simulink model "part2_MAIN_2019_ayonnn"  (R2023b)
settings: Solver=FixedStepAuto  StartTime=0.0  StopTime=8000  FixedStep=0.1  RelTol=1e-3
values from neighbouring files (symbols this model uses):
  Af = diag(ti)    [init.m]    (also in init_old.m)
  Aw = [zeros(3) eye(3) ... (first row only)    [get_observer_parameters.m]
  B = [thr1 thr2_x thr2_y thr3 thr4_x thr4_y thr5_x thr5_y]    [B_redistributed.m]    (also in check_alg.m = [1 2 3 4 5 6 7 8; get_observer_parameters.m = [zeros(6,3);zeros(3,3);zeros(3,3);inv(M)])
  change_position_time = 1200    [init.m]    (also in init_old.m)
  Cw = [zeros(3) eye(3)]    [get_observer_parameters.m]
  D = Damping    [init.m]    (also in init_old.m)
  Damping = diag([2.6486e5, 8.8164e5, 3.3774e8])    [init.m]    (also in init_old.m)
  direction_limit = pi/36    (= 0.0872664625997)    [init.m]    (also in init_old.m)
  direction_time_constant = 100    [init.m]    (also in init_old.m)
  dt = 0.1    [get_observer_parameters.m]
  E = [Ew, zeros(6,3) ... (first row only)    [get_observer_parameters.m]
  Gamma = diag(omega_is)    [init.m]    (also in init_old.m)
  gust_limit = 40    [init.m]    (also in init_old.m)
  H = [Cw, eye(3), zeros(3,3) zeros(3,3)]    [get_observer_parameters.m]    (also in quadprog.m = 2*diag([w.' w.' q.' q.' w_alpha.' w_alpha.']); quadprog_basic.m = 2*diag([w.' w.' q.' q.']); quadprog_false.m = 2*diag([w.' w.' q.' q.' w_alpha.' w_alpha.']))
  height = 3    [init.m]    (also in init_old.m)
  inv_M = inv(M)    [get_observer_parameters.m]
  inv_Tb = inv(Tb)    [get_observer_parameters.m]
  kappa = 0.003    [init.m]    (also in init_old.m)
  kappa2 = 0.0026    [init.m]    (also in init_old.m)
  Kd = [1660451.40544401; 3920391.80535684; 1605063439.04156]    [init.m]    (also in init_old.m)
  Ki = [137.081306245593; 3163.274947400198; 335358.448218978]    [init.m]    (also in init_old.m)
  Kp = [75459.3345349083; 277551.73586971; 120744473.878042]    [init.m]    (also in init_old.m)
  L = 1800    [init.m]    (also in init_old.m)
  M = Mass    [init.m]    (also in init_old.m)
  mean_wind_direction = pi    (= 3.14159265359)    [init.m]    (also in init_old.m)
  observer_type = 1    [init.m]    (also in init_old.m = 0)
  Omega = diag([omega_n, omega_n, omega_n])    [get_observer_parameters.m]    (also in init.m = diag(2*omega_is.*zeta_is); init_old.m = diag(2*omega_is.*zeta_is))
  Q = diag([0.1,0.1,pi/180,1e6,1e6,1e9])*10e3    [get_observer_parameters.m]
  R = diag([1,0.1,0.1*pi/180])*10e-3    [get_observer_parameters.m]
  simulation = 2    [init.m]    (also in init_old.m = 1)
  slow_varying_limit = 1    [init.m]    (also in init_old.m)
  slow_varying_time_constant = 100    [init.m]    (also in init_old.m)
  TAU = dt*E    [get_observer_parameters.m]
  Tb = 0.1 * eye(3)    [get_observer_parameters.m]
  u10 = 12    [init.m]    (also in init_old.m)
  vessel =     [test.mat]
  wind = 1    [init.m]    (also in init_old.m)
undefined symbols (not defined in the file or in its folder): Hoerner, ModelParams, npf, Param, thrusters, WaveModel
libraries: simulink x10, slpidlib x6, dspsigops x6, marine_hydro x4, marine_gnc x2
(part 2 of 3)

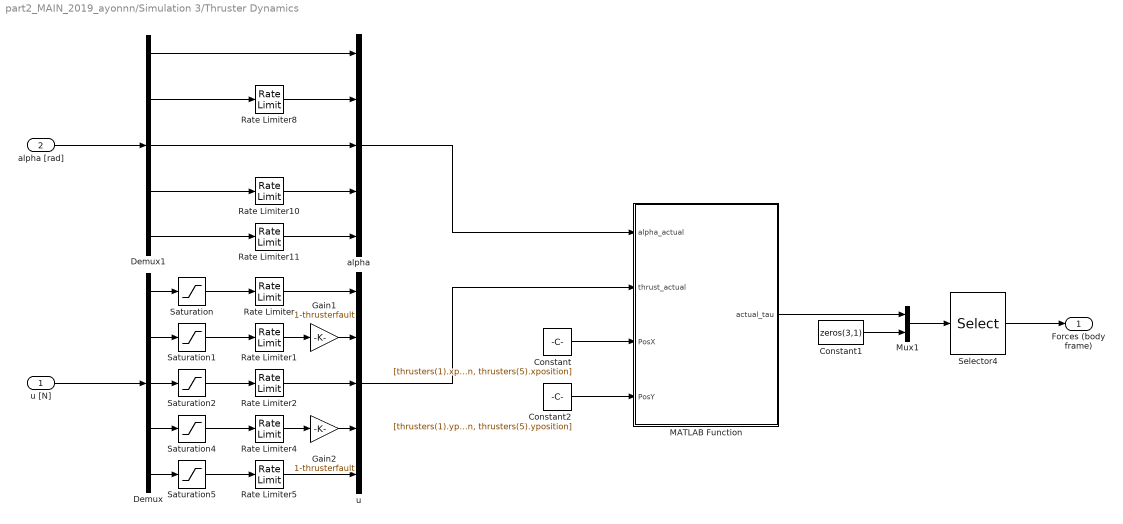
== system part2_MAIN_2019_ayonnn/Simulation 3/Thruster Dynamics ==
  u [N] : Inport
  alpha [rad] : Inport  Port=2
  Constant : Constant  Value=[thrusters(1).xposition, thrusters(2).xposition, thrusters(3).xposition, thrusters(4).xposition, thrusters(5).xposition]
  Constant1 : Constant  Value=zeros(3,1)
  Constant2 : Constant  Value=[thrusters(1).yposition, thrusters(2).yposition, thrusters(3).yposition, thrusters(4).yposition, thrusters(5).yposition]
  Demux : Demux  Outputs=5
  Demux1 : Demux  Outputs=5
  Gain1 : Gain  Gain=1-thrusterfault
  Gain2 : Gain  Gain=1-thrusterfault
  MATLAB Function : MATLAB Function  TreatAsAtomicUnit=on
  Mux1 : Mux  Inputs=2
  Rate Limiter : RateLimiter  RisingSlewLimit=thrusters(1).rate  FallingSlewLimit=-thrusters(1).rate  SampleTimeMode=inherited
  Rate Limiter1 : RateLimiter  RisingSlewLimit=thrusters(2).rate  FallingSlewLimit=-thrusters(2).rate  SampleTimeMode=inherited
  Rate Limiter10 : RateLimiter  RisingSlewLimit=thrusters(4).rotationspeed  FallingSlewLimit=-thrusters(4).rotationspeed  SampleTimeMode=inherited
  Rate Limiter11 : RateLimiter  RisingSlewLimit=thrusters(5).rotationspeed  FallingSlewLimit=-thrusters(5).rotationspeed  SampleTimeMode=inherited
  Rate Limiter2 : RateLimiter  RisingSlewLimit=thrusters(3).rate  FallingSlewLimit=-thrusters(3).rate  SampleTimeMode=inherited
  Rate Limiter4 : RateLimiter  RisingSlewLimit=thrusters(4).rate  FallingSlewLimit=-thrusters(4).rate  SampleTimeMode=inherited
  Rate Limiter5 : RateLimiter  RisingSlewLimit=thrusters(5).rate  FallingSlewLimit=-thrusters(5).rate  SampleTimeMode=inherited
  Rate Limiter8 : RateLimiter  RisingSlewLimit=thrusters(2).rotationspeed  FallingSlewLimit=-thrusters(2).rotationspeed  SampleTimeMode=inherited
  Saturation : Saturate  UpperLimit=thrusters(1).thrust  LowerLimit=-thrusters(1).thrust
  Saturation1 : Saturate  UpperLimit=thrusters(2).thrust  LowerLimit=-thrusters(2).thrust
  Saturation2 : Saturate  UpperLimit=thrusters(3).thrust  LowerLimit=-thrusters(3).thrust
  Saturation4 : Saturate  UpperLimit=thrusters(4).thrust  LowerLimit=-thrusters(4).thrust
  Saturation5 : Saturate  UpperLimit=thrusters(5).thrust  LowerLimit=-thrusters(5).thrust
  Selector4 : Selector  InputPortWidth=6  IndexOptions=Index vector (dialog)  Indices=[1 2 4 5 6 3]  OutputSizes=1
  alpha : Mux  Inputs=5
  u : Mux  Inputs=5
  "Forces (body frame) " : Outport  VectorParamsAs1DForOutWhenUnconnected=off
  wires:
  Rate Limiter2/1 -> u/3
  Saturation/1 -> Rate Limiter/1
  Mux1/1 -> Selector4/1
  Constant1/1 -> Mux1/2
  Saturation4/1 -> Rate Limiter4/1
  Demux/2 -> Saturation1/1
  Saturation1/1 -> Rate Limiter1/1
  Demux/1 -> Saturation/1
  Demux/3 -> Saturation2/1
  Saturation2/1 -> Rate Limiter2/1
  Selector4/1 -> "Forces (body frame) "/1
  Gain1/1 -> u/2
  Rate Limiter1/1 -> Gain1/1
  Rate Limiter/1 -> u/1
  Rate Limiter4/1 -> Gain2/1
  Saturation5/1 -> Rate Limiter5/1
  u [N]/1 -> Demux/1
  alpha [rad]/1 -> Demux1/1
  Constant/1 -> MATLAB Function/3(PosX)
  Constant2/1 -> MATLAB Function/4(PosY)
  u/1 -> MATLAB Function/2(thrust_actual)
  alpha/1 -> MATLAB Function/1(alpha_actual)
  MATLAB Function/1(actual_tau) -> Mux1/1
  Rate Limiter10/1 -> alpha/4
  Demux1/4 -> Rate Limiter10/1
  Demux1/5 -> Rate Limiter11/1
  Rate Limiter11/1 -> alpha/5
  Demux1/1 -> alpha/1
  Gain2/1 -> u/4
  Demux/4 -> Saturation4/1
  Demux/5 -> Saturation5/1
  Rate Limiter5/1 -> u/5
  Demux1/2 -> Rate Limiter8/1
  Rate Limiter8/1 -> alpha/2
  Demux1/3 -> alpha/3

== system part2_MAIN_2019_ayonnn/Simulation 3/Wave ==
  eta : Inport
  waves : Inport  Port=2
  Gain : Gain  Gain=waveforces
  Sum : Sum
  Wave loads (U=0) : marine_hydro/Hydro Library/Wave loads (U=0)  SystemSampleTime=-1  VariantActivationTime=update diagram  AllowFlexibleInterface=on  Latency=0  AutoFrameSizeCalculation=off
      settings: SourceProductName=MSS Hydro
  Wave : Outport  VectorParamsAs1DForOutWhenUnconnected=off
  wires:
  eta/1 -> Wave loads (U=0)/1
  waves/1 -> Wave loads (U=0)/2
  Sum/1 -> Gain/1
  Wave loads (U=0)/1 -> Sum/1
  Wave loads (U=0)/2 -> Sum/2
  Gain/1 -> Wave/1

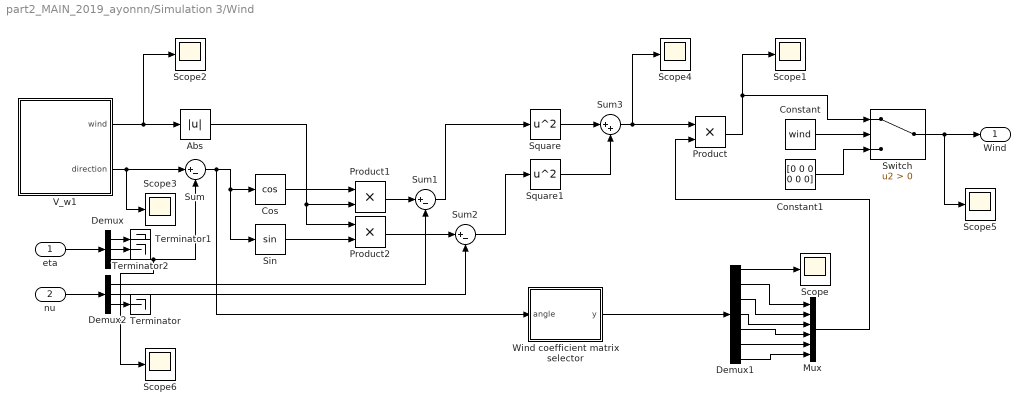
== system part2_MAIN_2019_ayonnn/Simulation 3/Wind ==
  eta : Inport
  nu : Inport  Port=2
  Abs : Abs  SaturateOnIntegerOverflow=off
  Constant : Constant  Value=wind
  Constant1 : Constant  Value=[0 0 0 0 0 0]
  Cos : Trigonometry  Operator=cos
  Demux : Demux  Outputs=3
  Demux1 : Demux  Outputs=7
  Demux2 : Demux  Outputs=3
  Mux : Mux  Inputs=6
  Product : Product
  Product1 : Product
  Product2 : Product
  Scope{,1..6} (7 alike) : Scope
  Sin : Trigonometry
  Square : Math  Operator=square  SignedPower=on
  Square1 : Math  Operator=square  SignedPower=on
  Sum : Sum  Inputs=|+-
  Sum1 : Sum  Inputs=|+-
  Sum2 : Sum  Inputs=|+-
  Sum3 : Sum  Inputs=|++
  Switch : Switch  Criteria=u2 > Threshold  SaturateOnIntegerOverflow=off  InputSameDT=off
  Terminator : Terminator
  Terminator1 : Terminator
  Terminator2 : Terminator
  V_w1 : Subsystem
  Wind coefficient matrix selector : MATLAB Function  TreatAsAtomicUnit=on
  Wind : Outport  VectorParamsAs1DForOutWhenUnconnected=off
  wires:
  V_w1/1(wind) -> Scope2/1, Abs/1
  Abs/1 -> Product2/1, Product1/2
  eta/1 -> Demux/1
  V_w1/2(direction) -> Scope3/1, Sum/1
  Demux/3 -> Scope6/1, Sum/2
  Wind coefficient matrix selector/1(y) -> Demux1/1
  Demux1/1 -> Scope/1
  Demux1/2 -> Mux/1
  Demux1/3 -> Mux/2
  Demux1/4 -> Mux/3
  Demux1/5 -> Mux/4
  Demux1/6 -> Mux/5
  Demux1/7 -> Mux/6
  Product/1 -> Switch/1, Scope1/1
  Mux/1 -> Product/2
  Sum/1 -> Wind coefficient matrix selector/1(angle), Sin/1, Cos/1
  nu/1 -> Demux2/1
  Sin/1 -> Product2/2
  Cos/1 -> Product1/1
  Product1/1 -> Sum1/1
  Product2/1 -> Sum2/1
  Demux2/1 -> Sum1/2
  Demux2/2 -> Sum2/2
  Sum1/1 -> Square/1
  Sum2/1 -> Square1/1
  Sum3/1 -> Scope4/1, Product/1
  Square/1 -> Sum3/1
  Square1/1 -> Sum3/2
  Demux2/3 -> Terminator/1
  Demux/1 -> Terminator1/1
  Demux/2 -> Terminator2/1
  Switch/1 -> Scope5/1, Wind/1
  Constant/1 -> Switch/2
  Constant1/1 -> Switch/3

== system part2_MAIN_2019_ayonnn/Original/Current (North - East)/Subsystem ==
  Mux1 : Mux  Inputs=3
  Scope : Scope
  Step1 : Step  Time=0  After=0  SampleTime=0
  Step2 : Step  Time=0  After=-0.2  SampleTime=0
  Step3 : Step  Time=0  After=0  SampleTime=0
  Out1 : Outport
  wires:
  Mux1/1 -> Scope/1, Out1/1
  Step1/1 -> Mux1/1
  Step2/1 -> Mux1/2
  Step3/1 -> Mux1/3

== system part2_MAIN_2019_ayonnn/Original/Current (North - East)/Subsystem1 ==
  Add : Sum  Inputs=+++
  Cos : Trigonometry  Operator=cos
  Gain : Gain  Gain=pi/180
  Matrix Multiply : Product
  Matrix Multiply1 : Product
  Mux : Mux  Inputs=3
  Ramp : simulink/Sources/Ramp  slope=0.45  start=2  InitialOutput=0
  Ramp1 : simulink/Sources/Ramp  slope=-0.45  start=202  InitialOutput=0
  Scope : Scope  NumInputPorts=3
  Sin : Trigonometry
  Step : Step  Time=2  After=0.5  SampleTime=0
  Step1 : Step  Time=2  Before=180  After=180  SampleTime=0
  Step2 : Step  Time=0  After=0  SampleTime=0
  Out1 : Outport
  wires:
  Step1/1 -> Add/1
  Ramp/1 -> Add/2
  Ramp1/1 -> Add/3
  Step/1 -> Matrix Multiply1/1, Matrix Multiply/1
  Sin/1 -> Matrix Multiply1/2, Scope/1
  Cos/1 -> Matrix Multiply/2, Scope/2
  Matrix Multiply/1 -> Mux/1
  Matrix Multiply1/1 -> Mux/2
  Step2/1 -> Mux/3
  Mux/1 -> Scope/3, Out1/1
  Add/1 -> Gain/1
  Gain/1 -> Sin/1, Cos/1

== system part2_MAIN_2019_ayonnn/Original/Current (North - East)/Subsystem2 ==
  Mux : Mux  Inputs=3
  Step : Step  Time=0  After=0  SampleTime=0
  Out1 : Outport
  wires:
  Mux/1 -> Out1/1
  Step/1 -> Mux/3, Mux/2, Mux/1

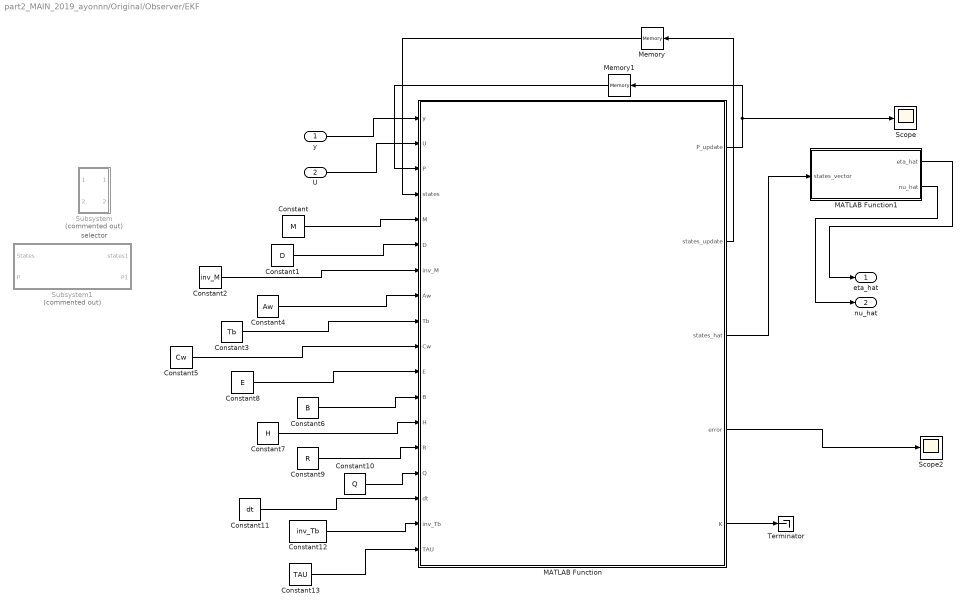
== system part2_MAIN_2019_ayonnn/Original/Observer/EKF ==
  note: selector
  y : Inport
  U : Inport  Port=2
  Constant : Constant  Value=M
  Constant1 : Constant  Value=D
  Constant10 : Constant  Value=Q
  Constant11 : Constant  Value=dt
  Constant12 : Constant  Value=inv_Tb
  Constant13 : Constant  Value=TAU
  Constant2 : Constant  Value=inv_M
  Constant3 : Constant  Value=Tb
  Constant4 : Constant  Value=Aw
  Constant5 : Constant  Value=Cw
  Constant6 : Constant  Value=B
  Constant7 : Constant  Value=H
  Constant8 : Constant  Value=E
  Constant9 : Constant  Value=R
  MATLAB Function : MATLAB Function  TreatAsAtomicUnit=on
  MATLAB Function1 : MATLAB Function  TreatAsAtomicUnit=on
  Memory : Memory  InitialCondition=zeros(15,1)
  Memory1 : Memory  InitialCondition=eye(15,15)
  Scope : Scope
  Scope2 : Scope
  Subsystem : Subsystem  Commented=on
  Subsystem1 : Subsystem  Commented=on
  Terminator : Terminator
  eta_hat : Outport
  nu_hat : Outport  Port=2
  wires:
  U/1 -> MATLAB Function/2(U)
  MATLAB Function1/1(eta_hat) -> eta_hat/1
  MATLAB Function/3(states_hat) -> MATLAB Function1/1(states_vector)
  MATLAB Function/4(error) -> Scope2/1
  y/1 -> MATLAB Function/1(y)
  MATLAB Function1/2(nu_hat) -> nu_hat/1
  MATLAB Function/2(states_update) -> Memory/1
  Constant/1 -> MATLAB Function/5(M)
  Constant1/1 -> MATLAB Function/6(D)
  Constant2/1 -> MATLAB Function/7(inv_M)
  Constant4/1 -> MATLAB Function/8(Aw)
  Constant3/1 -> MATLAB Function/9(Tb)
  Constant5/1 -> MATLAB Function/10(Cw)
  Constant8/1 -> MATLAB Function/11(E)
  Constant6/1 -> MATLAB Function/12(B)
  Constant7/1 -> MATLAB Function/13(H)
  Constant9/1 -> MATLAB Function/14(R)
  Constant10/1 -> MATLAB Function/15(Q)
  Constant11/1 -> MATLAB Function/16(dt)
  Constant12/1 -> MATLAB Function/17(inv_Tb)
  Constant13/1 -> MATLAB Function/18(TAU)
  Memory/1 -> MATLAB Function/4(states)
  MATLAB Function/1(P_update) -> Memory1/1, Scope/1
  Memory1/1 -> MATLAB Function/3(P)
  MATLAB Function/5(K) -> Terminator/1

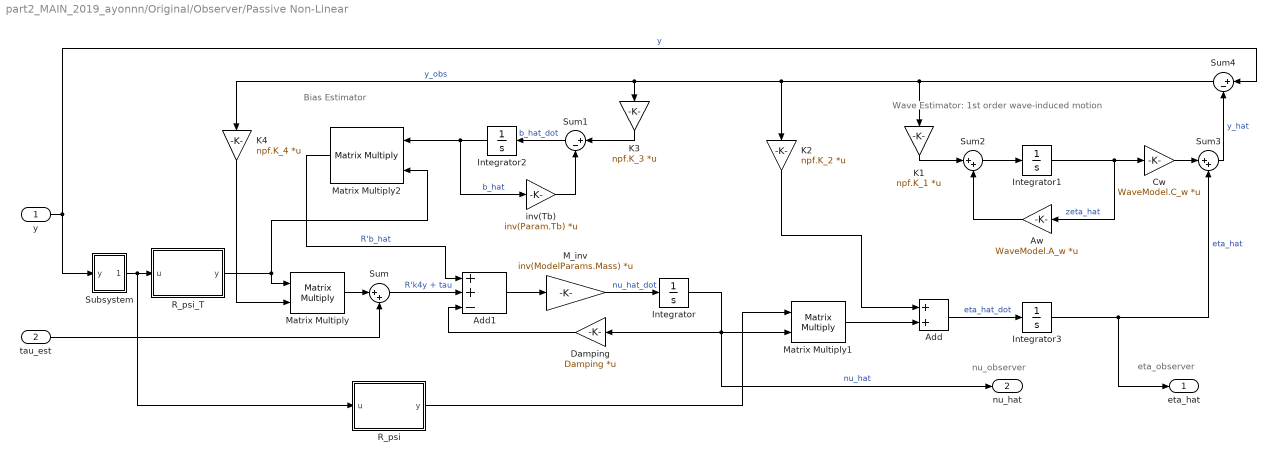
== system part2_MAIN_2019_ayonnn/Original/Observer/Passive Non-Linear ==
  note: eta_observer
  note: nu_observer
  note: Bias Estimator
  note: Wave Estimator: 1st order wave-induced motion
  y : Inport
  tau_est : Inport  Port=2
  Add : Sum
  Add1 : Sum  Inputs=++-
  Aw : Gain  Gain=WaveModel.A_w  Multiplication=Matrix(K*u)
  Cw : Gain  Gain=WaveModel.C_w  Multiplication=Matrix(K*u)
  Damping : Gain  Gain=Damping  Multiplication=Matrix(K*u)
  Integrator{,1..3} (4 alike) : Integrator
  K1 : Gain  Gain=npf.K_1  Multiplication=Matrix(K*u)
  K2 : Gain  Gain=npf.K_2  Multiplication=Matrix(K*u)
  K3 : Gain  Gain=npf.K_3  Multiplication=Matrix(K*u)
  K4 : Gain  Gain=npf.K_4  Multiplication=Matrix(K*u)
  M_inv : Gain  Gain=inv(ModelParams.Mass)  Multiplication=Matrix(K*u)
  Matrix Multiply : Product  Multiplication=Matrix(*)
  Matrix Multiply1 : Product  Multiplication=Matrix(*)
  Matrix Multiply2 : Product  Multiplication=Matrix(*)
  R_psi : MATLAB Function  TreatAsAtomicUnit=on
  R_psi_T : MATLAB Function  TreatAsAtomicUnit=on
  Subsystem : Subsystem
  Sum : Sum  Inputs=|++
  Sum1 : Sum  Inputs=|+-
  Sum2 : Sum  Inputs=|++
  Sum3 : Sum  Inputs=|++
  Sum4 : Sum  Inputs=|+-
  inv(Tb) : Gain  Gain=inv(Param.Tb)  Multiplication=Matrix(K*u)
  eta_hat : Outport
  nu_hat : Outport  Port=2
  wires:
  Matrix Multiply/1 -> Sum/1
  Matrix Multiply1/1 -> Add/2
  Matrix Multiply2/1 -> Add1/1  "R'b_hat"
  R_psi_T/1(y) -> Matrix Multiply/1, Matrix Multiply2/2
  Add1/1 -> M_inv/1
  Damping/1 -> Add1/3
  R_psi/1(y) -> Matrix Multiply1/1
  Sum/1 -> Add1/2  "R'k4y + tau"
  Add/1 -> Integrator3/1  "eta_hat_dot"
  inv(Tb)/1 -> Sum1/2
  y/1 -> Subsystem/1(y), Sum4/1  "y"
  Aw/1 -> Sum2/2
  K3/1 -> Sum1/1
  Cw/1 -> Sum3/1
  Integrator1/1 -> Cw/1, Aw/1  "zeta_hat"
  Sum1/1 -> Integrator2/1  "b_hat_dot"
  Integrator/1 -> nu_hat/1, Damping/1, Matrix Multiply1/2  "nu_hat"
  Sum4/1 -> K1/1, K2/1, K3/1, K4/1  "y_obs"
  Sum3/1 -> Sum4/2  "y_hat"
  Integrator3/1 -> eta_hat/1, Sum3/2  "eta_hat"
  Sum2/1 -> Integrator1/1
  K2/1 -> Add/1
  K4/1 -> Matrix Multiply/2
  M_inv/1 -> Integrator/1  "nu_hat_dot"
  Integrator2/1 -> inv(Tb)/1, Matrix Multiply2/1  "b_hat"
  tau_est/1 -> Sum/2
  K1/1 -> Sum2/1
  Subsystem/1(Out1) -> R_psi/1(u), R_psi_T/1(u)

== system part2_MAIN_2019_ayonnn/Original/Observer/Subsystem ==
  In1 : Inport
  Demux : Demux  Outputs=6
  Mux : Mux  Inputs=3
  Terminator : Terminator
  Terminator1 : Terminator
  Terminator2 : Terminator
  Out1 : Outport
  wires:
  Mux/1 -> Out1/1
  Demux/6 -> Mux/3
  Demux/5 -> Terminator2/1
  Demux/2 -> Mux/2
  Demux/1 -> Mux/1
  Demux/3 -> Terminator/1
  In1/1 -> Demux/1
  Demux/4 -> Terminator1/1

== system part2_MAIN_2019_ayonnn/Original/Reference Model/Simulation Selector ==
  note: simulation 1 and 2
  note: Simulation 4
  note: simulation 3
  Constant : Constant  Value=simulation
  Constant1 : Constant  Value=simulation
  Subsystem : Subsystem
  Subsystem1 : Subsystem
  Subsystem2 : Subsystem
  Switch : Switch  Criteria=u2 > Threshold  Threshold=3  SaturateOnIntegerOverflow=off  InputSameDT=off
  Switch1 : Switch  Criteria=u2 > Threshold  Threshold=2  SaturateOnIntegerOverflow=off  InputSameDT=off
  Out1 : Outport
  wires:
  Subsystem1/1(Out1) -> Switch/1
  Subsystem/1(Set-point) -> Switch/3
  Constant/1 -> Switch/2
  Switch/1 -> Switch1/1
  Constant1/1 -> Switch1/2
  Subsystem2/1(Out1) -> Switch1/3
  Switch1/1 -> Out1/1

== system part2_MAIN_2019_ayonnn/Original/Thrust Allocation/Unwrap ==
  alpha : Inport
  Demux : Demux  Outputs=5
  Mux : Mux  Inputs=5
  Unwrap : dspsigops/Unwrap  tol=pi  InputProcessing=Columns as channels (frame based)  running=off
  Unwrap1 : dspsigops/Unwrap  tol=pi  InputProcessing=Columns as channels (frame based)  running=off
  Unwrap2 : dspsigops/Unwrap  tol=pi  InputProcessing=Columns as channels (frame based)  running=off
  alpha [rad] : Outport
  wires:
  alpha/1 -> Demux/1
  Mux/1 -> alpha [rad]/1
  Demux/1 -> Mux/1
  Demux/4 -> Unwrap2/1
  Unwrap2/1 -> Mux/4
  Demux/5 -> Unwrap/1
  Unwrap/1 -> Mux/5
  Demux/3 -> Mux/3
  Demux/2 -> Unwrap1/1
  Unwrap1/1 -> Mux/2

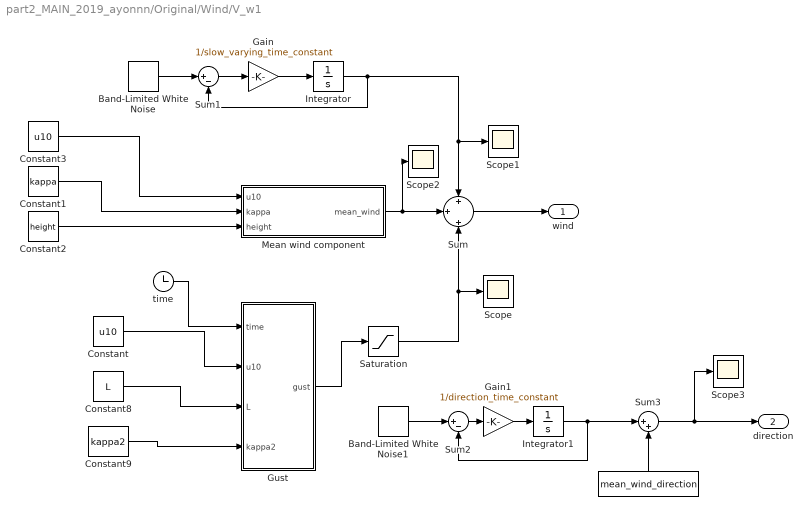
== system part2_MAIN_2019_ayonnn/Original/Wind/V_w1 ==
  " " : Constant  Value=mean_wind_direction
  Band-Limited White Noise : simulink/Sources/Band-Limited White Noise  Cov=np_slow_varying  Ts=0.1  seed=[23341]
  Band-Limited White Noise1 : simulink/Sources/Band-Limited White Noise  Cov=np_direction  Ts=0.1  seed=[23341]
  Constant : Constant  Value=u10
  Constant1 : Constant  Value=kappa
  Constant2 : Constant  Value=height
  Constant3 : Constant  Value=u10
  Constant8 : Constant  Value=L
  Constant9 : Constant  Value=kappa2
  Gain : Gain  Gain=1/slow_varying_time_constant
  Gain1 : Gain  Gain=1/direction_time_constant
  Gust : MATLAB Function  TreatAsAtomicUnit=on
  Integrator : Integrator  LimitOutput=on  UpperSaturationLimit=slow_varying_limit  LowerSaturationLimit=-slow_varying_limit
  Integrator1 : Integrator  LimitOutput=on  UpperSaturationLimit=direction_limit  LowerSaturationLimit=-direction_limit
  Mean wind component : MATLAB Function  TreatAsAtomicUnit=on
  Saturation : Saturate  UpperLimit=gust_limit  LowerLimit=-10
  Scope{,1..3} (4 alike) : Scope
  Sum : Sum  Inputs=+|+|+
  Sum1 : Sum  Inputs=|+-
  Sum2 : Sum  Inputs=|+-
  Sum3 : Sum  Inputs=|++
  time : Clock
  wind : Outport
  direction : Outport  Port=2
  wires:
  Constant3/1 -> Mean wind component/1(u10)
  Constant1/1 -> Mean wind component/2(kappa)
  Constant2/1 -> Mean wind component/3(height)
  Mean wind component/1(mean_wind) -> Scope2/1, Sum/2
  Sum/1 -> wind/1
  Integrator/1 -> Scope1/1, Sum/1, Sum1/2
  Band-Limited White Noise/1 -> Sum1/1
  Integrator1/1 -> Sum2/2, Sum3/1
  Band-Limited White Noise1/1 -> Sum2/1
  " "/1 -> Sum3/2
  Sum3/1 -> Scope3/1, direction/1
  Gain1/1 -> Integrator1/1
  Sum2/1 -> Gain1/1
  Gain/1 -> Integrator/1
  Sum1/1 -> Gain/1
  Constant8/1 -> Gust/3(L)
  Gust/1(gust) -> Saturation/1
  Saturation/1 -> Sum/3, Scope/1
  Constant9/1 -> Gust/4(kappa2)
  Constant/1 -> Gust/2(u10)
  time/1 -> Gust/1(time)

== system part2_MAIN_2019_ayonnn/Simulation 3/Current (North - East)/Subsystem ==
  Mux1 : Mux  Inputs=3
  Scope : Scope
  Step1 : Step  Time=0  After=0  SampleTime=0
  Step2 : Step  Time=0  After=-0.2  SampleTime=0
  Step3 : Step  Time=0  After=0  SampleTime=0
  Out1 : Outport
  wires:
  Mux1/1 -> Scope/1, Out1/1
  Step1/1 -> Mux1/1
  Step2/1 -> Mux1/2
  Step3/1 -> Mux1/3

== system part2_MAIN_2019_ayonnn/Simulation 3/Current (North - East)/Subsystem1 ==
  Add : Sum  Inputs=+++
  Cos : Trigonometry  Operator=cos
  Gain : Gain  Gain=pi/180
  Matrix Multiply : Product
  Matrix Multiply1 : Product
  Mux : Mux  Inputs=3
  Ramp : simulink/Sources/Ramp  slope=0.45  start=2  InitialOutput=0
  Ramp1 : simulink/Sources/Ramp  slope=-0.45  start=202  InitialOutput=0
  Scope : Scope  NumInputPorts=3
  Sin : Trigonometry
  Step : Step  Time=2  After=0.5  SampleTime=0
  Step1 : Step  Time=2  Before=180  After=180  SampleTime=0
  Step2 : Step  Time=0  After=0  SampleTime=0
  Out1 : Outport
  wires:
  Step1/1 -> Add/1
  Ramp/1 -> Add/2
  Ramp1/1 -> Add/3
  Step/1 -> Matrix Multiply1/1, Matrix Multiply/1
  Sin/1 -> Matrix Multiply1/2, Scope/1
  Cos/1 -> Matrix Multiply/2, Scope/2
  Matrix Multiply/1 -> Mux/1
  Matrix Multiply1/1 -> Mux/2
  Step2/1 -> Mux/3
  Mux/1 -> Scope/3, Out1/1
  Add/1 -> Gain/1
  Gain/1 -> Sin/1, Cos/1

== system part2_MAIN_2019_ayonnn/Simulation 3/Current (North - East)/Subsystem2 ==
  Mux : Mux  Inputs=3
  Step : Step  Time=0  After=0  SampleTime=0
  Out1 : Outport
  wires:
  Mux/1 -> Out1/1
  Step/1 -> Mux/3, Mux/2, Mux/1

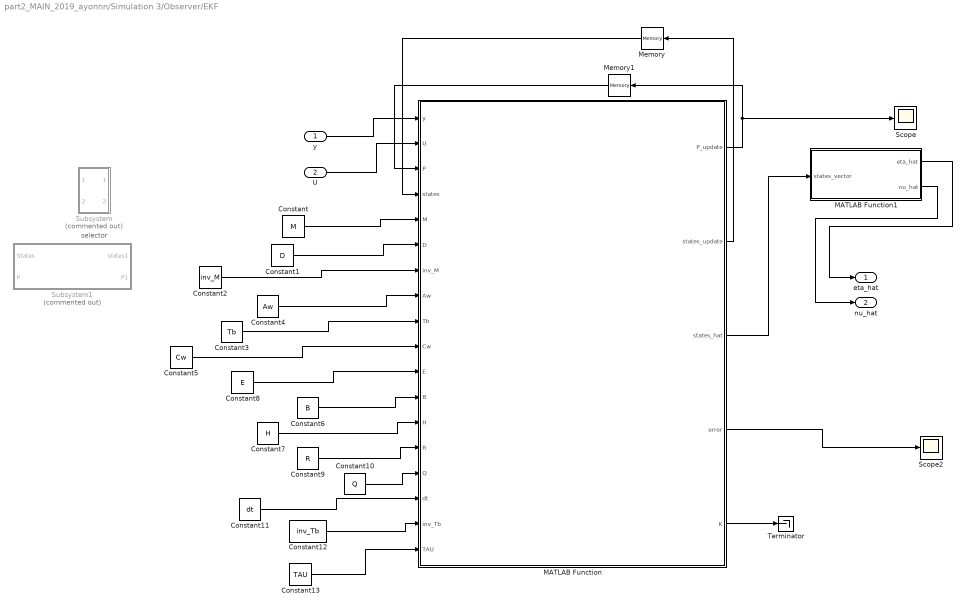
== system part2_MAIN_2019_ayonnn/Simulation 3/Observer/EKF ==
  note: selector
  y : Inport
  U : Inport  Port=2
  Constant : Constant  Value=M
  Constant1 : Constant  Value=D
  Constant10 : Constant  Value=Q
  Constant11 : Constant  Value=dt
  Constant12 : Constant  Value=inv_Tb
  Constant13 : Constant  Value=TAU
  Constant2 : Constant  Value=inv_M
  Constant3 : Constant  Value=Tb
  Constant4 : Constant  Value=Aw
  Constant5 : Constant  Value=Cw
  Constant6 : Constant  Value=B
  Constant7 : Constant  Value=H
  Constant8 : Constant  Value=E
  Constant9 : Constant  Value=R
  MATLAB Function : MATLAB Function  TreatAsAtomicUnit=on
  MATLAB Function1 : MATLAB Function  TreatAsAtomicUnit=on
  Memory : Memory  InitialCondition=zeros(15,1)
  Memory1 : Memory  InitialCondition=eye(15,15)
  Scope : Scope
  Scope2 : Scope
  Subsystem : Subsystem  Commented=on
  Subsystem1 : Subsystem  Commented=on
  Terminator : Terminator
  eta_hat : Outport
  nu_hat : Outport  Port=2
  wires:
  U/1 -> MATLAB Function/2(U)
  MATLAB Function1/1(eta_hat) -> eta_hat/1
  MATLAB Function/3(states_hat) -> MATLAB Function1/1(states_vector)
  MATLAB Function/4(error) -> Scope2/1
  y/1 -> MATLAB Function/1(y)
  MATLAB Function1/2(nu_hat) -> nu_hat/1
  MATLAB Function/2(states_update) -> Memory/1
  Constant/1 -> MATLAB Function/5(M)
  Constant1/1 -> MATLAB Function/6(D)
  Constant2/1 -> MATLAB Function/7(inv_M)
  Constant4/1 -> MATLAB Function/8(Aw)
  Constant3/1 -> MATLAB Function/9(Tb)
  Constant5/1 -> MATLAB Function/10(Cw)
  Constant8/1 -> MATLAB Function/11(E)
  Constant6/1 -> MATLAB Function/12(B)
  Constant7/1 -> MATLAB Function/13(H)
  Constant9/1 -> MATLAB Function/14(R)
  Constant10/1 -> MATLAB Function/15(Q)
  Constant11/1 -> MATLAB Function/16(dt)
  Constant12/1 -> MATLAB Function/17(inv_Tb)
  Constant13/1 -> MATLAB Function/18(TAU)
  Memory/1 -> MATLAB Function/4(states)
  MATLAB Function/1(P_update) -> Memory1/1, Scope/1
  Memory1/1 -> MATLAB Function/3(P)
  MATLAB Function/5(K) -> Terminator/1

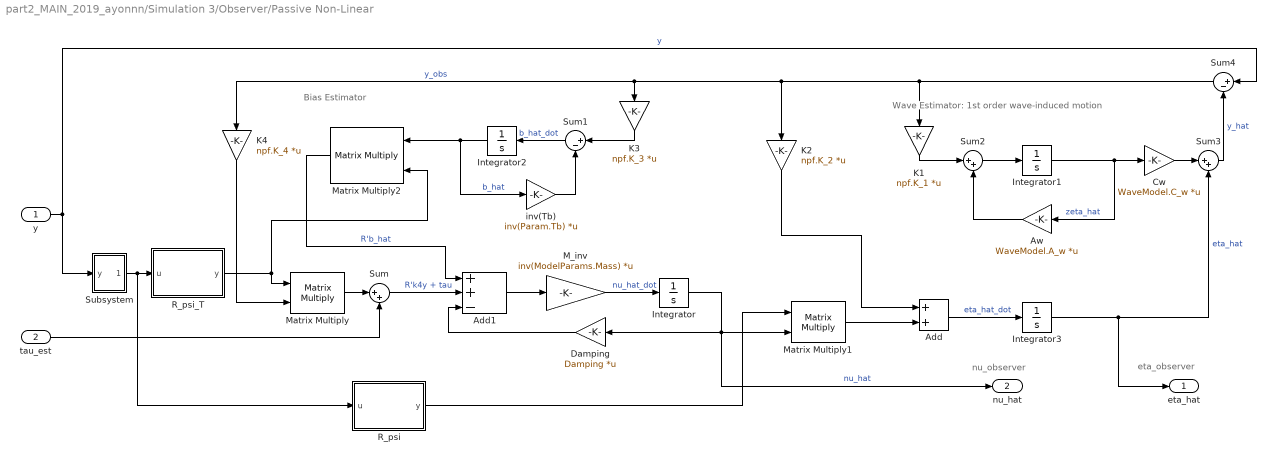
== system part2_MAIN_2019_ayonnn/Simulation 3/Observer/Passive Non-Linear ==
  note: eta_observer
  note: nu_observer
  note: Bias Estimator
  note: Wave Estimator: 1st order wave-induced motion
  y : Inport
  tau_est : Inport  Port=2
  Add : Sum
  Add1 : Sum  Inputs=++-
  Aw : Gain  Gain=WaveModel.A_w  Multiplication=Matrix(K*u)
  Cw : Gain  Gain=WaveModel.C_w  Multiplication=Matrix(K*u)
  Damping : Gain  Gain=Damping  Multiplication=Matrix(K*u)
  Integrator{,1..3} (4 alike) : Integrator
  K1 : Gain  Gain=npf.K_1  Multiplication=Matrix(K*u)
  K2 : Gain  Gain=npf.K_2  Multiplication=Matrix(K*u)
  K3 : Gain  Gain=npf.K_3  Multiplication=Matrix(K*u)
  K4 : Gain  Gain=npf.K_4  Multiplication=Matrix(K*u)
  M_inv : Gain  Gain=inv(ModelParams.Mass)  Multiplication=Matrix(K*u)
  Matrix Multiply : Product  Multiplication=Matrix(*)
  Matrix Multiply1 : Product  Multiplication=Matrix(*)
  Matrix Multiply2 : Product  Multiplication=Matrix(*)
  R_psi : MATLAB Function  TreatAsAtomicUnit=on
  R_psi_T : MATLAB Function  TreatAsAtomicUnit=on
  Subsystem : Subsystem
  Sum : Sum  Inputs=|++
  Sum1 : Sum  Inputs=|+-
  Sum2 : Sum  Inputs=|++
  Sum3 : Sum  Inputs=|++
  Sum4 : Sum  Inputs=|+-
  inv(Tb) : Gain  Gain=inv(Param.Tb)  Multiplication=Matrix(K*u)
  eta_hat : Outport
  nu_hat : Outport  Port=2
  wires:
  Matrix Multiply/1 -> Sum/1
  Matrix Multiply1/1 -> Add/2
  Matrix Multiply2/1 -> Add1/1  "R'b_hat"
  R_psi_T/1(y) -> Matrix Multiply/1, Matrix Multiply2/2
  Add1/1 -> M_inv/1
  Damping/1 -> Add1/3
  R_psi/1(y) -> Matrix Multiply1/1
  Sum/1 -> Add1/2  "R'k4y + tau"
  Add/1 -> Integrator3/1  "eta_hat_dot"
  inv(Tb)/1 -> Sum1/2
  y/1 -> Subsystem/1(y), Sum4/1  "y"
  Aw/1 -> Sum2/2
  K3/1 -> Sum1/1
  Cw/1 -> Sum3/1
  Integrator1/1 -> Cw/1, Aw/1  "zeta_hat"
  Sum1/1 -> Integrator2/1  "b_hat_dot"
  Integrator/1 -> nu_hat/1, Damping/1, Matrix Multiply1/2  "nu_hat"
  Sum4/1 -> K1/1, K2/1, K3/1, K4/1  "y_obs"
  Sum3/1 -> Sum4/2  "y_hat"
  Integrator3/1 -> eta_hat/1, Sum3/2  "eta_hat"
  Sum2/1 -> Integrator1/1
  K2/1 -> Add/1
  K4/1 -> Matrix Multiply/2
  M_inv/1 -> Integrator/1  "nu_hat_dot"
  Integrator2/1 -> inv(Tb)/1, Matrix Multiply2/1  "b_hat"
  tau_est/1 -> Sum/2
  K1/1 -> Sum2/1
  Subsystem/1(Out1) -> R_psi/1(u), R_psi_T/1(u)

== system part2_MAIN_2019_ayonnn/Simulation 3/Observer/Subsystem ==
  In1 : Inport
  Demux : Demux  Outputs=6
  Mux : Mux  Inputs=3
  Terminator : Terminator
  Terminator1 : Terminator
  Terminator2 : Terminator
  Out1 : Outport
  wires:
  Mux/1 -> Out1/1
  Demux/6 -> Mux/3
  Demux/5 -> Terminator2/1
  Demux/2 -> Mux/2
  Demux/1 -> Mux/1
  Demux/3 -> Terminator/1
  In1/1 -> Demux/1
  Demux/4 -> Terminator1/1

== system part2_MAIN_2019_ayonnn/Simulation 3/Reference Model/Simulation Selector ==
  Simulation 1 : Subsystem
  Simulation 2 : Subsystem
  Out1 : Outport
  wires:
  Simulation 2/1(Out1) -> Out1/1

== system part2_MAIN_2019_ayonnn/Simulation 3/Thrust Allocation/Unwrap ==
  alpha : Inport
  Demux : Demux  Outputs=5
  Mux : Mux  Inputs=5
  Unwrap : dspsigops/Unwrap  tol=pi  InputProcessing=Columns as channels (frame based)  running=off
  Unwrap1 : dspsigops/Unwrap  tol=pi  InputProcessing=Columns as channels (frame based)  running=off
  Unwrap2 : dspsigops/Unwrap  tol=pi  InputProcessing=Columns as channels (frame based)  running=off
  alpha [rad] : Outport
  wires:
  alpha/1 -> Demux/1
  Mux/1 -> alpha [rad]/1
  Demux/1 -> Mux/1
  Demux/4 -> Unwrap2/1
  Unwrap2/1 -> Mux/4
  Demux/5 -> Unwrap/1
  Unwrap/1 -> Mux/5
  Demux/3 -> Mux/3
  Demux/2 -> Unwrap1/1
  Unwrap1/1 -> Mux/2

== system part2_MAIN_2019_ayonnn/Simulation 3/Wind/V_w1 ==
  " " : Constant  Value=mean_wind_direction
  Band-Limited White Noise : simulink/Sources/Band-Limited White Noise  Cov=np_slow_varying  Ts=0.1  seed=[23341]
  Band-Limited White Noise1 : simulink/Sources/Band-Limited White Noise  Cov=np_direction  Ts=0.1  seed=[23341]
  Constant : Constant  Value=u10
  Constant1 : Constant  Value=kappa
  Constant2 : Constant  Value=height
  Constant3 : Constant  Value=u10
  Constant8 : Constant  Value=L
  Constant9 : Constant  Value=kappa2
  Gain : Gain  Gain=1/slow_varying_time_constant
  Gain1 : Gain  Gain=1/direction_time_constant
  Gust : MATLAB Function  TreatAsAtomicUnit=on
  Integrator : Integrator  LimitOutput=on  UpperSaturationLimit=slow_varying_limit  LowerSaturationLimit=-slow_varying_limit
  Integrator1 : Integrator  LimitOutput=on  UpperSaturationLimit=direction_limit  LowerSaturationLimit=-direction_limit
  Mean wind component : MATLAB Function  TreatAsAtomicUnit=on
  Saturation : Saturate  UpperLimit=gust_limit  LowerLimit=-10
  Scope{,1..3} (4 alike) : Scope
  Sum : Sum  Inputs=+|+|+
  Sum1 : Sum  Inputs=|+-
  Sum2 : Sum  Inputs=|+-
  Sum3 : Sum  Inputs=|++
  time : Clock
  wind : Outport
  direction : Outport  Port=2
  wires:
  Constant3/1 -> Mean wind component/1(u10)
  Constant1/1 -> Mean wind component/2(kappa)
  Constant2/1 -> Mean wind component/3(height)
  Mean wind component/1(mean_wind) -> Scope2/1, Sum/2
  Sum/1 -> wind/1
  Integrator/1 -> Scope1/1, Sum/1, Sum1/2
  Band-Limited White Noise/1 -> Sum1/1
  Integrator1/1 -> Sum2/2, Sum3/1
  Band-Limited White Noise1/1 -> Sum2/1
  " "/1 -> Sum3/2
  Sum3/1 -> Scope3/1, direction/1
  Gain1/1 -> Integrator1/1
  Sum2/1 -> Gain1/1
  Gain/1 -> Integrator/1
  Sum1/1 -> Gain/1
  Constant8/1 -> Gust/3(L)
  Gust/1(gust) -> Saturation/1
  Saturation/1 -> Sum/3, Scope/1
  Constant9/1 -> Gust/4(kappa2)
  Constant/1 -> Gust/2(u10)
  time/1 -> Gust/1(time)

== system part2_MAIN_2019_ayonnn/Original/Observer/EKF/Subsystem ==
  note: simulation time
  note: P_selector
  In1 : Inport
  In2 : Inport  Port=2
  Constant1 : Constant  Value=eye(15)
  Constant2 : Constant  Value=zeros(15,1)
  Step : Step  Time=0.01  SampleTime=0.1
  Switch : Switch  Threshold=1  SaturateOnIntegerOverflow=off  InputSameDT=off
  Switch1 : Switch  Threshold=1  SaturateOnIntegerOverflow=off  InputSameDT=off
  Out1 : Outport
  Out2 : Outport  Port=2
  wires:
  Switch1/1 -> Out2/1
  In1/1 -> Switch/1
  In2/1 -> Switch1/1
  Switch/1 -> Out1/1
  Constant1/1 -> Switch/3
  Step/1 -> Switch1/2, Switch/2
  Constant2/1 -> Switch1/3

== system part2_MAIN_2019_ayonnn/Original/Observer/EKF/Subsystem1 ==
  note: P
  note: states
  note: simulation time
  States : Inport
  P : Inport  Port=2
  MATLAB Function : MATLAB Function  TreatAsAtomicUnit=on
  Step1 : Step  Time=0.01  After=10  SampleTime=0.1
  states1 : Outport
  P1 : Outport  Port=2
  wires:
  Step1/1 -> MATLAB Function/1(u)
  P/1 -> MATLAB Function/2(P)
  States/1 -> MATLAB Function/3(states)
  MATLAB Function/1(P1) -> P1/1
  MATLAB Function/2(states1) -> states1/1

== system part2_MAIN_2019_ayonnn/Original/Observer/Passive Non-Linear/Subsystem ==
  y : Inport
  Demux : Demux  Outputs=3
  Terminator : Terminator
  Terminator1 : Terminator
  Out1 : Outport
  wires:
  y/1 -> Demux/1
  Demux/3 -> Out1/1
  Demux/1 -> Terminator/1
  Demux/2 -> Terminator1/1

== system part2_MAIN_2019_ayonnn/Original/Reference Model/Simulation Selector/Subsystem ==
  note: yaw
  note: sway
  note: surge
  Mux : Mux  Inputs=3
  Scope : Scope
  Step : Step  After=10  SampleTime=0
  Step1 : Step  After=10  SampleTime=0
  Step2 : Step  After=3*pi/2  SampleTime=0
  Set-point : Outport
  wires:
  Step/1 -> Mux/1
  Step1/1 -> Mux/2
  Step2/1 -> Mux/3
  Mux/1 -> Scope/1, Set-point/1

== system part2_MAIN_2019_ayonnn/Original/Reference Model/Simulation Selector/Subsystem1 ==
  note: yaw
  note: sway
  note: surge
  Add : Sum
  Add1 : Sum
  Add2 : Sum
  Mux : Mux  Inputs=3
  Scope : Scope
  Step : Step  Time=10  After=50  SampleTime=0
  Step1 : Step  Time=change_position_time  After=-50  SampleTime=0
  Step2 : Step  Time=change_position_time*2  After=pi/4  SampleTime=0
  Step3 : Step  Time=change_position_time*3  After=-50  SampleTime=0
  Step4 : Step  Time=change_position_time*4  After=50  SampleTime=0
  Step5 : Step  Time=change_position_time*4  After=-pi/4  SampleTime=0
  Out1 : Outport
  wires:
  Mux/1 -> Scope/1, Out1/1
  Step/1 -> Add/1
  Step3/1 -> Add/2
  Step1/1 -> Add1/1
  Step4/1 -> Add1/2
  Step2/1 -> Add2/1
  Step5/1 -> Add2/2
  Add/1 -> Mux/1
  Add1/1 -> Mux/2
  Add2/1 -> Mux/3

== system part2_MAIN_2019_ayonnn/Original/Reference Model/Simulation Selector/Subsystem2 ==
  Mux : Mux  Inputs=3
  Step : Step  After=0  SampleTime=0
  Step1 : Step  After=0  SampleTime=0
  Step2 : Step  After=0  SampleTime=0
  Out1 : Outport
  wires:
  Step/1 -> Mux/1
  Step1/1 -> Mux/2
  Step2/1 -> Mux/3
  Mux/1 -> Out1/1

== system part2_MAIN_2019_ayonnn/Simulation 3/Observer/EKF/Subsystem ==
  note: simulation time
  note: P_selector
  In1 : Inport
  In2 : Inport  Port=2
  Constant1 : Constant  Value=eye(15)
  Constant2 : Constant  Value=zeros(15,1)
  Step : Step  Time=0.01  SampleTime=0.1
  Switch : Switch  Threshold=1  SaturateOnIntegerOverflow=off  InputSameDT=off
  Switch1 : Switch  Threshold=1  SaturateOnIntegerOverflow=off  InputSameDT=off
  Out1 : Outport
  Out2 : Outport  Port=2
  wires:
  Switch1/1 -> Out2/1
  In1/1 -> Switch/1
  In2/1 -> Switch1/1
  Switch/1 -> Out1/1
  Constant1/1 -> Switch/3
  Step/1 -> Switch1/2, Switch/2
  Constant2/1 -> Switch1/3

== system part2_MAIN_2019_ayonnn/Simulation 3/Observer/EKF/Subsystem1 ==
  note: P
  note: states
  note: simulation time
  States : Inport
  P : Inport  Port=2
  MATLAB Function : MATLAB Function  TreatAsAtomicUnit=on
  Step1 : Step  Time=0.01  After=10  SampleTime=0.1
  states1 : Outport
  P1 : Outport  Port=2
  wires:
  Step1/1 -> MATLAB Function/1(u)
  P/1 -> MATLAB Function/2(P)
  States/1 -> MATLAB Function/3(states)
  MATLAB Function/1(P1) -> P1/1
  MATLAB Function/2(states1) -> states1/1

== system part2_MAIN_2019_ayonnn/Simulation 3/Observer/Passive Non-Linear/Subsystem ==
  y : Inport
  Demux : Demux  Outputs=3
  Terminator : Terminator
  Terminator1 : Terminator
  Out1 : Outport
  wires:
  y/1 -> Demux/1
  Demux/3 -> Out1/1
  Demux/1 -> Terminator/1
  Demux/2 -> Terminator1/1

== system part2_MAIN_2019_ayonnn/Simulation 3/Reference Model/Simulation Selector/Simulation 1 ==
  note: yaw
  note: sway
  note: surge
  Mux : Mux  Inputs=3
  Ramp : simulink/Sources/Ramp  slope=1  start=0  InitialOutput=0
  Saturation : Saturate
  Scope : Scope
  Step : Step  Time=0  After=0  SampleTime=0
  Step1 : Step  Time=change_position_time  After=0  SampleTime=0
  Step2 : Step  Time=change_position_time*2  After=0  SampleTime=0
  Step3 : Step  Time=change_position_time*3  After=-50  SampleTime=0
  Step4 : Step  Time=change_position_time*4  After=50  SampleTime=0
  Step5 : Step  Time=change_position_time*4  After=-pi/4  SampleTime=0
  Out1 : Outport
  wires:
  Mux/1 -> Scope/1, Out1/1
  Step3/1 -> ?
  Step1/1 -> Mux/2
  Step4/1 -> ?
  Step2/1 -> Mux/3
  Step5/1 -> ?
  Step/1 -> Mux/1
  Ramp/1 -> Saturation/1

== system part2_MAIN_2019_ayonnn/Simulation 3/Reference Model/Simulation Selector/Simulation 2 ==
  note: yaw
  note: sway
  note: surge
  Add : Sum
  Add1 : Sum
  Add2 : Sum
  Mux : Mux  Inputs=3
  Ramp : simulink/Sources/Ramp  slope=1  start=0  InitialOutput=0
  Saturation : Saturate
  Scope : Scope
  Step : Step  Time=0  After=50  SampleTime=0
  Step1 : Step  Time=change_position_time  After=-50  SampleTime=0
  Step2 : Step  Time=change_position_time*2  After=pi/4  SampleTime=0
  Step3 : Step  Time=change_position_time*3  After=-50  SampleTime=0
  Step4 : Step  Time=change_position_time*4  After=50  SampleTime=0
  Step5 : Step  Time=change_position_time*4  After=-pi/4  SampleTime=0
  Out1 : Outport
  wires:
  Mux/1 -> Scope/1, Out1/1
  Step/1 -> Add/1
  Step3/1 -> Add/2
  Step1/1 -> Add1/1
  Step4/1 -> Add1/2
  Step2/1 -> Add2/1
  Step5/1 -> Add2/2
  Add/1 -> Mux/1
  Add1/1 -> Mux/2
  Add2/1 -> Mux/3
  Ramp/1 -> Saturation/1

== matlab function part2_MAIN_2019_ayonnn/Original/Observer/EKF/MATLAB Function1 ==
  data: states_vector input; eta_hat output; nu_hat output
function [eta_hat, nu_hat] = fcn(states_vector)
%%states [zeta,eta, b, nu] --15x1
%zeta - 6x1, 
%eta - 3x1, 
%b - 3x1, 
%nu - 3x1
eta_hat = states_vector(7:9,1);
nu_hat = states_vector(13:15,1);

end

== matlab function part2_MAIN_2019_ayonnn/Original/Wind/V_w1/Gust ==
  settings: updateMethod=DISCRETE
  data: time input; u10 input; L input; kappa2 input; gust output
function gust = fcn(time, u10, L, kappa2)

nfreq = 100;
phases = 2*pi * rand(nfreq,1);
gust_tot = 0;
f = zeros(1, nfreq);

for i = 1:nfreq
    f(i) = 0.01 + (i-1)/(nfreq-1) * 0.99;
    f_tilde = L*f(i)/u10;
    S = (4*kappa2*L*u10)/((2+f_tilde^2)^(5/6));
    df = abs(f(2) - f(1));
    gust_part = sqrt(2*S*df)*cos(2*pi*f(i)*time + phases(i));
    gust_tot = gust_tot + gust_part;
end

gust = gust_tot;

== matlab function part2_MAIN_2019_ayonnn/Original/Wind/V_w1/Mean wind component ==
  data: u10 input; mean_wind output; kappa input; height input
function mean_wind = fcn(u10, kappa, height)
z0 = 10*exp(-2/(5*sqrt(kappa)));
mean_wind = u10 * (5/2) * sqrt(kappa)*log(height/z0);

== matlab function part2_MAIN_2019_ayonnn/Original/Observer/EKF/Subsystem1/MATLAB Function ==
  data: u input; P1 output; P input; states input; states1 output
function [P1, states1] = fcn(u, P, states)

if u>1
    P1 = eye(15);
    states1 = zeros(15,1);
else
    P1 = P;
    states1 = states;
end

== matlab function part2_MAIN_2019_ayonnn/Simulation 3/Current (North - East)/MATLAB Function ==
  data: u input; y output
function y = fcn(u)
rot = [cos(u) -sin(u) 0;
    sin(u) cos(u) 0;
    0 0 1];

y = rot';

== matlab function part2_MAIN_2019_ayonnn/Original/Thrust Allocation/MATLAB Function1 ==
  data: tau_d input; Td output; alpha output
function [Td, alpha] = quad_prog_basic_slow(tau_d)
%% x, y, and psi component of tau_d
tau = [tau_d(1); tau_d(2); tau_d(6)]; 

%% Quadratic Programming
% Compute function arguments
% Point to Minimize
u_p = [0 0 0 0 0 0 0 0].'; % [T1 T2x T2y T3 T4x T4y T5x T5y]
u_m = -[0 0 0 0 0 0 0 0].'; % [T1 T2x T2y T3 T4x T4y T5x T5y]
s_p = [0 0 0].'; % [x1 x2 x6]
s_m = -[0 0 0].'; % [x1 x2 x6]
x0 = [u_p; u_m; s_p; s_m]; % auxiliary variables

% persistent x0_l
% 
% % Store previous point
% if isempty(x0_l)
%     x0_l = x0(1:16);
% end

% Objective Function
% Quadratic Objective Term
sWeight = 1e4;
w = [1 1 1 1 0.8 0.8 0.8 0.8]; % Prioritize control over T4 and T5
q = [sWeight sWeight sWeight*10]; % For slackness (Needs Tuning)
H = 2*diag([w w q q]);

% Linear Objective Term
% f = zeros(1, length(x0)); % No linear term in the objective function
f = [];

% Thruster Equality Constraints
% Thruster 1
x1 = 39.3;
y1 = 0;
% Thruster 2
x2 = 35.6;
y2 = 0;
% Thruster 3
x3 = 31.3;
y3 = 0;
% Thruster 4
x4 = -28.5;
y4 = 5;
% Thruster 5
x5 = -28.5;
y5 = -5;

% Redistributed force for each thruster
thr1 = [0 1 x1].';
thr2_x = [1 0 y2].';
thr2_y = [0 1 x2].';
thr3 = [0 1 x3].';
thr4_x = [1 0 y4].';
thr4_y = [0 1 x4].';
thr5_x = [1 0 y5].';
thr5_y = [0 1 x5].';

% B redistributed
B_r = [thr1 thr2_x thr2_y thr3 thr4_x thr4_y thr5_x thr5_y];

Aeq = [B_r -B_r eye(3) -eye(3)];
beq = tau;

% Thruster Saturation Constraints
u_max = [125000, 150000, 150000, 125000, 300000, 300000, 300000, 300000].';
% u_min = [-125000 0 0 -125000 0 0 0 0].';
u_min = -u_max;

% Rate Limitation Constraints
timestep = 0.1;
delta_max = [125000/8*timestep, 150000/8*timestep, 150000/8*timestep, 125000/8*timestep, 300000/10*timestep, 300000/10*timestep, 300000/10*timestep, 300000/10*timestep];
delta_min = -delta_max;

% lim_max = delta_max - x0_l;
% lim_min = delta_min + x0_l;

A = [eye(8) -eye(8) zeros(8,3) zeros(8,3);
     -eye(8) eye(8) zeros(8,3) zeros(8,3)];

% b = [-(max(u_min, lim_min));
%      min(u_max, lim_max)];
b = [-u_min;
    u_max];

lb = [];
ub = [];

options = optimoptions('quadprog', 'Algorithm', 'active-set');

% Compute optimal thruster control
x0_opt = quadprog(H,f,A,b,Aeq,beq,lb,ub,x0, options);

% % Store previous x0_opt
% x0_l = x0_opt(1:16);

% Slack Variable from auxiliary variables
s = x0_opt(17:19) - x0_opt(20:22); % STILL DON'T NOW WHAT TO DO WITH THIS
s_abs = x0_opt(17:19) + x0_opt(20:22); % STILL DON'T NOW WHAT TO DO WITH THIS

% Allocation variables from auxiliary variables
u = x0_opt(1:8) - x0_opt(9:16); 
u_abs = x0_opt(1:8) + x0_opt(9:16); 

%% RESULTS
% Thruster control
Td = [u(1); 
      sqrt(u(2)^2 + u(3)^2); 
      u(4); 
      sqrt(u(5)^2 + u(6)^2);
      sqrt(u(7)^2 + u(8)^2)];

% Thruster angle
alpha2 = atan2(u(3),u(2));
alpha4 = atan2(u(6),u(5));
alpha5 = atan2(u(8),u(7));
alpha = [pi/2; alpha2; pi/2; alpha4; alpha5];
end
% function [Td, alpha] = quad_prog_basic(tau_d)
% %% x, y, and psi component of tau_d
% tau = [tau_d(1); tau_d(2); tau_d(6)]; 
% 
% %% Quadratic Programming
% % Compute function arguments
% % Point to Minimize
% u = [0 0 0 0 0 0 0 0].'; % [T1 T2x T2y T3 T4x T4y T5x T5y]
% s = [0 0 0].'; % [x1 x2 x6]
% x0 = [u; s]; % auxiliary variables
% 
% % persistent x0_l
% % 
% % if isempty(x0_l)
% %     x0_l = x0;
% % end
% 
% % Objective Function
% % Quadratic Objective Term
% sWeight = 1e4;
% w = [1 1 1 1 0.8 0.8 0.8 0.8]; % Prioritize control over T4 and T5
% q = [sWeight sWeight sWeight*10]; % For slackness (Needs Tuning)
% H = 2*diag([w q]);
% 
% % Linear Objective Term
% f = zeros(length(x0),1); % No linear term in the objective function 
% % f = [];
% 
% % Thruster Equality Constraints
% % Thruster 1
% x1 = 39.3;
% y1 = 0;
% % Thruster 2
% x2 = 35.6;
% y2 = 0;
% % Thruster 3
% x3 = 31.3;
% y3 = 0;
% % Thruster 4
% x4 = -28.5;
% y4 = 5;
% % Thruster 5
% x5 = -28.5;
% y5 = -5;
% 
% % Redistributed force for each thruster
% thr1 = [0 1 x1].';
% thr2_x = [1 0 y2].';
% thr2_y = [0 1 x2].';
% thr3 = [0 1 x3].';
% thr4_x = [1 0 y4].';
% thr4_y = [0 1 x4].';
% thr5_x = [1 0 y5].';
% thr5_y = [0 1 x5].';
% 
% % B redistributed
% B_r = [thr1 thr2_x thr2_y thr3 thr4_x thr4_y thr5_x thr5_y];
% 
% Aeq = [B_r, -eye(3)];
% beq = tau;
% 
% % Thruster Saturation Constraints
% u_max = [125000 150000 150000 125000 300000 300000 300000 300000].';
% u_min = -u_max;
% % u_min = [-125000 0 0 -125000 0 0 0 0].';
% 
% A = [-eye(8), zeros(8,3);
%      eye(8), zeros(8,3)];
% 
% b = [-u_min;
%      u_max];
% 
% % coder.extrinsic('quadprog');
% % coder.extrinsic('optimoptions');
% % options = optimoptions('quadprog','Algorithm','interior-point-convex','Display','off','Steptolerance',1e-30,'OptimalityTolerance',1e+3);
% options = optimoptions('quadprog', 'Algorithm', 'active-set');
% % options = optimoptions('quadprog', 'Algorithm', 'interior-point-convex', 'Display', 'iter');
% 
% % Compute optimal thruster control\
% x0_opt = quadprog(H,f,A,b,Aeq,beq,[],[],x0,options);
% 
% % Store previous x0_opt
% % x0_l = x0_opt;
% 
% % Allocation variables from auxiliary variables
% u_f = x0_opt(1:8); 
% 
% %% RESULTS
% % Thruster control
% Td = [u_f(1); 
%       sqrt(u_f(2)^2 + u_f(3)^2); 
%       u_f(4); 
%       sqrt(u_f(5)^2 + u_f(6)^2);
%       sqrt(u_f(7)^2 + u_f(8)^2)];
% 
% % Thruster angle
% alpha2 = atan2(u_f(3),u_f(2));
% alpha4 = atan2(u_f(6),u_f(5));
% alpha5 = atan2(u_f(8),u_f(7));
% alpha = [pi/2; alpha2; pi/2; alpha4; alpha5];
% end

== matlab function part2_MAIN_2019_ayonnn/Original/Thrust Allocation/MATLAB Function2 ==
  data: tau_d input; Td output; alpha output
function [Td, alpha] = p_inv_B_S(tau_d)
%% Build the B matrix
% Thruster 1
x1 = 39.3;
y1 = 0;
% Thruster 2
x2 = 35.6;
y2 = 0;
% Thruster 3
x3 = 31.3;
y3 = 0;
% Thruster 4
x4 = -28.5;
y4 = 5;
% Thruster 5
x5 = -28.5;
y5 = -5;

% Redistributed force for each thruster
thr1 = [0 1 x1].';
thr2_x = [1 0 y2].';
thr2_y = [0 1 x2].';
thr3 = [0 1 x3].';
thr4_x = [1 0 y4].';
thr4_y = [0 1 x4].';
thr5_x = [1 0 y5].';
thr5_y = [0 1 x5].';

% B redistributed
B = [thr1 thr2_x thr2_y thr3 thr4_x thr4_y thr5_x thr5_y];

%% Result
tau = [tau_d(1); tau_d(2); tau_d(6)];

Td_r = pinv(B) * tau;

% Thruster control
Td = [Td_r(1); 
      sqrt(Td_r(2)^2 + Td_r(3)^2); 
      Td_r(4); 
      sqrt(Td_r(5)^2 + Td_r(6)^2);
      sqrt(Td_r(7)^2 + Td_r(8)^2)];

alpha2 = atan2(Td_r(3),Td_r(2));
alpha4 = atan2(Td_r(6),Td_r(5));
alpha5 = atan2(Td_r(8),Td_r(7));

alpha = [pi/2; alpha2; pi/2; alpha4; alpha5];

%% Saturation limit constraint
% Azimuth thruster
Td_max = [125000; 150000; 125000; 300000; 300000];
Td_min = [-125000; 0; -125000; 0; 0]; 

azimuth = [2; 4; 5];

% Find the indices of elements in u that are greater than their respective 
% elements in u_max
ind_remove = find(Td > Td_max | Td < Td_min);
ind_keep = find(Td < Td_max & Td > Td_min);

% Apply new constraint, don't change if thruster control didn't go above
% the constraints
if length(ind_remove) == length(Td)
    Td(Td > Td_max) = Td_max(Td > Td_max);
    Td(Td < Td_min) = Td_min(Td < Td_min);
elseif length(ind_remove) ~= length(Td_min) && ~isempty(ind_remove)
    % Use ismember to check if the azimuth outside the constraint
    isInArray = sum(ismember(azimuth, ind_remove));

    % Count how many thruster outside the constraint
    count_remove = length(ind_remove) + isInArray;

    % Create new_B and with new dimension
    new_B = zeros(3, size(B,2)-count_remove);

    % Go over the keeped column
    k = 1;
    for i = 1:length(ind_keep)
        % Computing the new_B
        if ind_keep(i) == 1
            new_B(:,k) = B(:, 1);
            k = k + 1;
        elseif ind_keep(i) == 2
            new_B(:,k:(k+1)) = B(:, 2:3);
            k = k + 2;
        elseif ind_keep(i) == 3
            new_B(:,k) = B(:, 4);
            k = k + 1;
        elseif ind_keep(i) == 4
            new_B(:,k:(k+1)) = B(:, 5:6);
            k = k + 2;
        elseif ind_keep(i) == 5
            new_B(:,k:(k+1)) = B(:, 7:8);
            k = k + 2;
        end 
    end

    % Compute the new_tau with a reduction from the maximum thruster
    new_tau = tau;
    for i = 1:length(ind_remove)
        if ind_remove(i) == 1
            new_tau = new_tau - (B(:,1)*Td_r(1));
        elseif ind_remove(i) == 2
            new_tau = new_tau - sqrt((B(:,2)*Td_r(2)).^2 +(B(:,3)*Td_r(3)).^2);
        elseif ind_remove(i) == 3
            new_tau = new_tau - (B(:,3)*Td_r(4));
        elseif ind_remove(i) == 4
            new_tau = new_tau - sqrt((B(:,5)*Td_r(5)).^2 +(B(:,6)*Td_r(6)).^2);
        elseif ind_remove(i) == 5
            new_tau = new_tau - sqrt((B(:,7)*Td_r(7)).^2 +(B(:,8)*Td_r(8)).^2);
        end
    end
    
    % Compute new_Td_r
    new_Td_i = pinv(new_B) * new_tau;

    % % Compute new_Td
    new_Td_r = zeros(length(Td_r),1);
     
    for i = 1:length(ind_remove)
        if ind_remove(i) == 1
            new_Td_r(1) = Td_r(1);
        elseif ind_remove(i) == 2
            new_Td_r(2:3) = Td_r(2:3);
        elseif ind_remove(i) == 3
            new_Td_r(4) = Td_r(4);
        elseif ind_remove(i) == 4
            new_Td_r(5:6) = Td_r(5:6);
        elseif ind_remove(i) == 5
            new_Td_r(7:8) = Td_r(7:8);
        end
    end

    k = 1;
    for i = 1:length(ind_keep)
        if ind_keep(i) == 1
            new_Td_r(1) = new_Td_i(k);
            k = k+1;
        elseif ind_keep(i) == 2
            new_Td_r(2:3) = new_Td_i(k:(k+1));
            k = k+2;
        elseif ind_keep(i) == 3
            new_Td_r(4) = new_Td_i(k);
            k = k+1;
        elseif ind_keep(i) == 4
            new_Td_r(5:6) = new_Td_i(k:(k+1));
            k = k+2;
        elseif ind_keep(i) == 5
            new_Td_r(7:8) = new_Td_i(k:(k+1));
            k = k+2;
        end
    end
    Td_r = new_Td_r;
    Td = [Td_r(1); 
          sqrt(Td_r(2)^2 + Td_r(3)^2); 
          Td_r(4); 
          sqrt(Td_r(5)^2 + Td_r(6)^2);
          sqrt(Td_r(7)^2 + Td_r(8)^2)];

    alpha2 = atan2(Td_r(3),Td_r(2));
    alpha4 = atan2(Td_r(6),Td_r(5));
    alpha5 = atan2(Td_r(8),Td_r(7));

    alpha = [pi/2; alpha2; pi/2; alpha4; alpha5];
end

== matlab function part2_MAIN_2019_ayonnn/Original/Wind/Wind coefficient matrix selector ==
  data: y output; angle input
function y = fcn(angle)

wind_coeff = [
  0  248.3700 0 0 0 -2355.232759 0
 10  265.1900 61.332 0 275.994 -2514.732759 551.1
 20  224.1300 136.22 0 612.99 -2125.37069 661.56
 30  149.0300 238.76 0 1074.42 -1413.215517 451.37
 40  134.3600 319.42 0 1437.39 -1274.103448 212.51
 50   96.8000 380.5 0 1712.25 -917.9310345 -23.578
 60   41.3640 396.1 0 1782.45 -392.2448276 1168.3
 70   16.4770 372.96 0 1678.32 -156.2474138 2376.3
 80    0.30412 376.5 0 1694.25 -2.883896552 3511.9
 90   -3.7230 390.01 0 1755.045 35.30431034 4610.4
100  -24.8790 386.63 0 1739.835 235.9215517 4769.5
110  -61.2810 393.76 0 1771.92 581.112931 5921.9
120 -108.5000 408.66 0 1838.97 1028.87931 6542.8
130 -169.3500 393.26 0 1769.67 1605.905172 6805.2
140 -206.6300 276.93 0 1246.185 1959.422414 6751.5
150 -201.9900 200.64 0 902.88 1915.422414 6190.1
160 -196.5100 124.71 0 561.195 1863.456897 3758.8
170 -181.5300 56.27 0 253.215 1721.405172 1905.6
180 -208.2200 0 0 0 1974.5 0
190 -181.5300 -56.27 0 -253.215 1721.405172 -1905.6
200 -196.5100 -124.71 0 -561.195 1863.456897 -3758.8
210 -201.9900 -200.64 0 -902.88 1915.422414 -6190.1
220 -206.6300 -276.93 0 -1246.185 1959.422414 -6751.5
230 -169.3500 -393.26 0 -1769.67 1605.905172 -6805.2
240 -108.5000 -408.66 0 -1838.97 1028.87931 -6542.8
250  -61.2810 -393.76 0 -1771.92 581.112931 -5921.9
260  -24.8790 -386.63 0 -1739.835 235.9215517 -4769.5
270  -3.72300 -390.01 0 -1755.045 35.30431034 -4610.4
280   0.30412 -376.5 0 -1694.25 -2.883896552 -3511.9
290  16.47700 -372.96 0 -1678.32 -156.2474138 -2376.3
300  41.36400 -396.1 0 -1782.45 -392.2448276 -1168.3
310  96.80000 -380.5 0 -1712.25 -917.9310345 23.578
320  134.3600 -319.42 0 -1437.39 -1274.103448 -212.51
330  149.0300 -238.76 0 -1074.42 -1413.215517 -451.37
340  224.1300 -136.22 0 -612.99 -2125.37069 -661.56
350  265.1900 -61.332 0 -275.994 -2514.732759 -551.1
360  248.3700 0 0 0 -2355.232759 0];

angle = abs(angle);

angle = (180/pi)*angle;

if angle > 360
    angle = angle - 360;
end



angle = int32(angle);

angle = int32(10*floor(angle/10));

i = 1;
j = 1;

while j < 38
    if int32(wind_coeff(j,1)) == angle
        i = j;
    end
    j = j+1;
end
y = wind_coeff(i,:);
